simulink model "Modelo_2_tanques"  (R2020b)
settings: Solver=ode45  StartTime=0.0  StopTime=100  RelTol=1e-3  EnableMultiTasking=on
settings Model: Creator=admin  LastModifiedBy=Marce
settings DataIOCC: LimitDataPoints=on  SaveFormat=Array  SignalLoggingSaveFormat=ModelDataLogs  ReturnWorkspaceOutputs=off
settings OptimizationCC: ExpressionDepthLimit=2147483647  LifeSpan=inf
settings DebuggingCC: UnderspecifiedInitializationDetection=Classic  MergeDetectMultiDrivingBlocksExec=none  SolverPrmCheckMsg=warning  FcnCallInpInsideContextMsg=warning  StateNameClashWarn=warning  SFUnexpectedBacktrackingDiag=warning  SFNoUnconditionalDefaultTransitionDiag=warning  SFExecutionAtInitializationDiag=none  ArithmeticOperatorsInVariantConditions=warning
settings HardwareCC: ProdBitPerPointer=32  ProdBitPerSizeT=32  ProdBitPerPtrDiffT=32  ProdLargestAtomicFloat=None  ProdIntDivRoundTo=Undefined  ProdEndianess=Unspecified  ProdWordSize=32  ProdHWDeviceType=32-bit Generic
settings ModelReferenceCC: PropagateSignalLabelsOutOfModel=off
settings SFSimCC: SimUseLocalCustomCode=off  CustomCodeUndefinedFunction=UseInterfaceOnly
settings RTWCC: RTWUseLocalCustomCode=off
settings CodeAppCC: StateflowObjectComments=on
settings GRTTargetCC: TargetLangStandard=C89/C90 (ANSI)  CombineOutputUpdateFcns=off  GRTInterface=on
settings ConfigComp: CovMetricSettings=dw  CovSaveCumulativeToWorkspaceVar=on  CovSaveSingleToWorkspaceVar=on  CovExternalEMLEnable=off

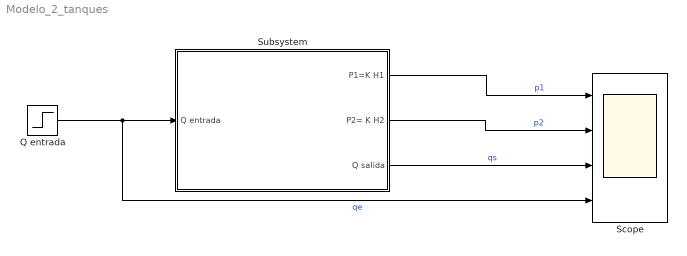
== system Modelo_2_tanques ==
  Q entrada : Step  After=10  SampleTime=0
  Scope : Scope  NumInputPorts=4
  Subsystem : Subsystem  mask(Sistema de dos tanques){Ch1=10, R1=1, Ch2=10, R2=1}
      mask prompts: Ch1 "Capacidad del tanque 1"; R1 "Restriccion para el tanque 1"; Ch2 "Capacidad del tanque 2"; R2 "Restriccion para el tanque 2"
  wires:
  Q entrada/1 -> Scope/4, Subsystem/1(Q entrada)  "qe"
  Subsystem/3(Q salida) -> Scope/3  "qs"
  Subsystem/1(P1=K H1) -> Scope/1  "p1"
  Subsystem/2(P2= K H2) -> Scope/2  "p2"

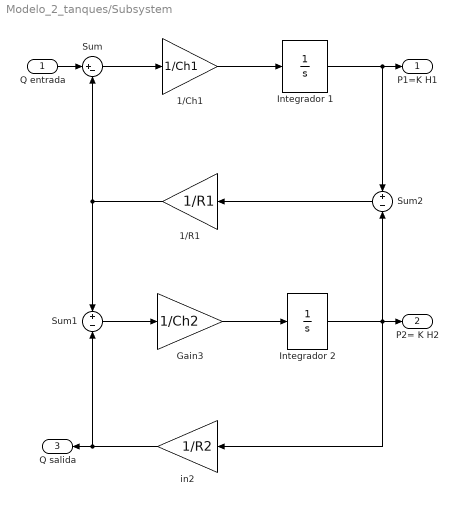
== system Modelo_2_tanques/Subsystem ==
  Q entrada : Inport
  1/Ch1 : Gain  Gain=1/Ch1
  1/R1 : Gain  Gain=1/R1
  Gain3 : Gain  Gain=1/Ch2
  Integrador 1 : Integrator
  Integrador 2 : Integrator
  Sum : Sum  Inputs=|+-
  Sum1 : Sum  Inputs=+|-
  Sum2 : Sum  Inputs=+|-
  in2 : Gain  Gain=1/R2
  P1=K H1 : Outport
  P2= K H2 : Outport  Port=2
  Q salida : Outport  Port=3
  wires:
  Sum/1 -> 1/Ch1/1
  1/Ch1/1 -> Integrador 1/1
  Sum2/1 -> 1/R1/1
  Sum1/1 -> Gain3/1
  Gain3/1 -> Integrador 2/1
  1/R1/1 -> Sum1/1, Sum/2
  in2/1 -> Sum1/2, Q salida/1
  Integrador 1/1 -> Sum2/1, P1=K H1/1
  Integrador 2/1 -> Sum2/2, P2= K H2/1, in2/1
  Q entrada/1 -> Sum/1
